simulink model "Demo_01_sim"  (R2018b)
settings: Solver=ode45  StartTime=0.0  StopTime=td  FixedStep=Tc  MaxStep=Tc  RelTol=1e-8  AbsTol=1e-8
values from neighbouring files (symbols this model uses):
  Gv = 12/5    (= 2.4)    [Demo_01.m]    (also in Demo_02.m = 3.63636363636; Demo_03.m = 3.63636363636; Demo_03b.m = 3.63636363636; Demo_04.m)
  km = 1/Kb    [Demo_01.m]    (also in Demo_02.m; Demo_03.m; Demo_03b.m; Demo_04.m)
  Kp = 0.02    [Demo_01.m]    (also in Demo_02.m; Demo_03.m = 0.1; Demo_03b.m = 5; Demo_04.m = 0.1)
  Kt = 0.0052226    [parametros_motor_25D.m]    (also in parametros_motor_37D.m = 0.0055601)
  Ra = 8.751992253    [parametros_motor_25D.m]    (also in parametros_motor_37D.m = 4.952082603)
  th_ref = 1    [Demo_01.m]    (also in Demo_03.m; Demo_03b.m; Demo_05.m; Demo_07.m)
  TL = 5*0.01    (= 0.05)    [Demo_01.m]    (also in Demo_02.m = 0; Demo_03.m = 0; Demo_03b.m = 0; Demo_04.m = 0)
  Tm = (Ra*Jm)/(Kb*Kt)    [Demo_01.m]    (also in Demo_02.m; Demo_03.m; Demo_03b.m; Demo_04.m)
  Tp = 100    [Demo_01.m]    (also in Demo_02.m; Demo_03.m = 10; Demo_03b.m = 10; Demo_04.m = 10)
  Ts = 0.001    [Control_optimo.m]    (also in Demo_01.m; Demo_02.m; Demo_03.m; Demo_03b.m)
settings Model: ExtModeAutoUpdateStatusClock=off  Creator=luigivillani  LastModifiedBy=Ivan
settings SolverCC: AutoScaleAbsTol=off  InitialStep=0.1*Tc
settings DataIOCC: SaveFormat=Array  SignalLoggingSaveFormat=ModelDataLogs  SaveOutput=off  SaveTime=off
settings OptimizationCC: BlockReduction=off  BooleanDataType=off  ExpressionDepthLimit=2147483647  InitFltsAndDblsToZero=on  LifeSpan=inf
settings DebuggingCC: SaveWithParameterizedLinksMsg=none  UnderspecifiedInitializationDetection=Classic  MergeDetectMultiDrivingBlocksExec=none  SignalResolutionControl=TryResolveAllWithWarning  MultiTaskDSMMsg=warning  MultiTaskCondExecSysMsg=none  FcnCallInpInsideContextMsg=warning  StateNameClashWarn=warning  SFUnexpectedBacktrackingDiag=warning  SFNoUnconditionalDefaultTransitionDiag=warning  SFExecutionAtInitializationDiag=none
settings HardwareCC: ProdBitPerPointer=32  ProdBitPerSizeT=32  ProdBitPerPtrDiffT=32  ProdLargestAtomicFloat=None  ProdIntDivRoundTo=Undefined  ProdEndianess=Unspecified  ProdWordSize=32  ProdHWDeviceType=32-bit Generic  TargetUnknown=on
settings ModelReferenceCC: PropagateSignalLabelsOutOfModel=off
settings CodeAppCC: StateflowObjectComments=on
settings GRTTargetCC: TargetFcnLib=ansi_tfl_tmw.mat  TargetLangStandard=C89/C90 (ANSI)  CombineOutputUpdateFcns=off  GRTInterface=on
settings ConfigComp: CovMetricSettings=dw  CovHtmlReporting=on  CovSaveCumulativeToWorkspaceVar=on  CovSaveSingleToWorkspaceVar=on

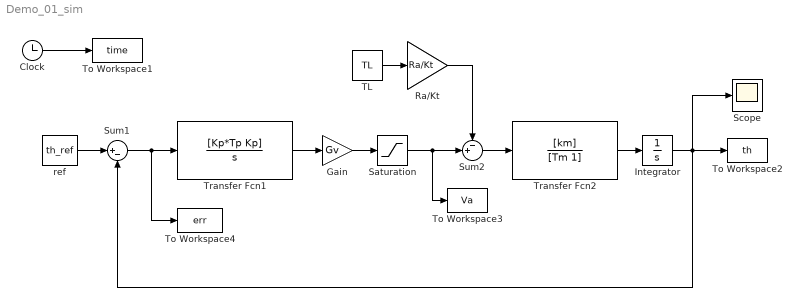
== system Demo_01_sim ==
  Clock : Clock
  Gain : Gain  Gain=Gv
  Integrator : Integrator
  Ra/Kt : Gain  Gain=Ra/Kt
  Saturation : Saturate  UpperLimit=12  LowerLimit=-12
  Scope : Scope
  Sum1 : Sum  Inputs=|+-  SaturateOnIntegerOverflow=on  InputSameDT=on  OutDataTypeStr=Inherit: Same as first input
  Sum2 : Sum  Inputs=-+|  SaturateOnIntegerOverflow=on  InputSameDT=on  OutDataTypeStr=Inherit: Same as first input
  TL : Constant  Value=TL
  To Workspace1 : ToWorkspace  VariableName=time  SampleTime=Ts
      settings: MaxDataPoints=ceil(td/Tc)
  To Workspace2 : ToWorkspace  VariableName=th  SampleTime=Ts
      settings: MaxDataPoints=ceil(td/Tc)
  To Workspace3 : ToWorkspace  VariableName=Va  SampleTime=Ts
      settings: MaxDataPoints=ceil(td/Tc)
  To Workspace4 : ToWorkspace  VariableName=err  SampleTime=Ts
      settings: MaxDataPoints=ceil(td/Tc)
  Transfer Fcn1 : TransferFcn  Numerator=[Kp*Tp Kp]  Denominator=[1 0]
  Transfer Fcn2 : TransferFcn  Numerator=[km]  Denominator=[Tm 1]
  ref : Constant  Value=th_ref
  wires:
  Clock/1 -> To Workspace1/1
  Transfer Fcn2/1 -> Integrator/1
  Sum2/1 -> Transfer Fcn2/1
  Ra/Kt/1 -> Sum2/1
  TL/1 -> Ra/Kt/1
  Transfer Fcn1/1 -> Gain/1
  ref/1 -> Sum1/1
  Integrator/1 -> Scope/1, To Workspace2/1, Sum1/2
  Sum1/1 -> Transfer Fcn1/1, To Workspace4/1
  Gain/1 -> Saturation/1
  Saturation/1 -> To Workspace3/1, Sum2/2
